simulink model "main_simulation"  (R2022b)
settings: Solver=VariableStepAuto  StartTime=0  StopTime=1372  FixedStep=0.1  MaxStep=0.1  RelTol=1e-3
values from neighbouring files (symbols this model uses):
  T = T(1:length(T)-100)    [data_loader.m]
libraries: spsVoltageMeasurementLib x2, spsControlledVoltageSourceLib x2, spsPMSynchronousMachineModel x1, simulink x1, autolibshared x1, slpidlib x1, spsStairGeneratorLib x1, spspowerguiLib x1
settings Model: Creator=Ahmad Hussain Safder  LastModifiedBy=safder.1
settings SolverCC: ZeroCrossAlgorithm=Adaptive
settings DataIOCC: SaveOutput=off  SaveTime=off  ReturnWorkspaceOutputs=off
settings DebuggingCC: IgnoredZcDiagnostic=none  UnconnectedInputMsg=warning  UnconnectedOutputMsg=warning  UnconnectedLineMsg=warning  ArithmeticOperatorsInVariantConditions=warning
settings ModelReferenceCC: EnableRefExpFcnMdlSchedulingChecks=on
settings SFSimCC: CustomCodeUndefinedFunction=UseInterfaceOnly

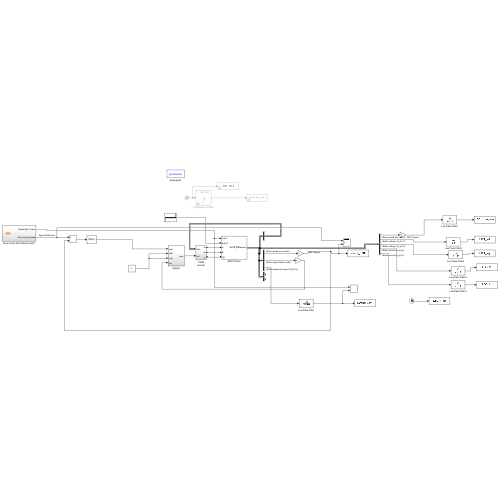
[thumbnail: Simulink's stored preview of the top-level diagram]
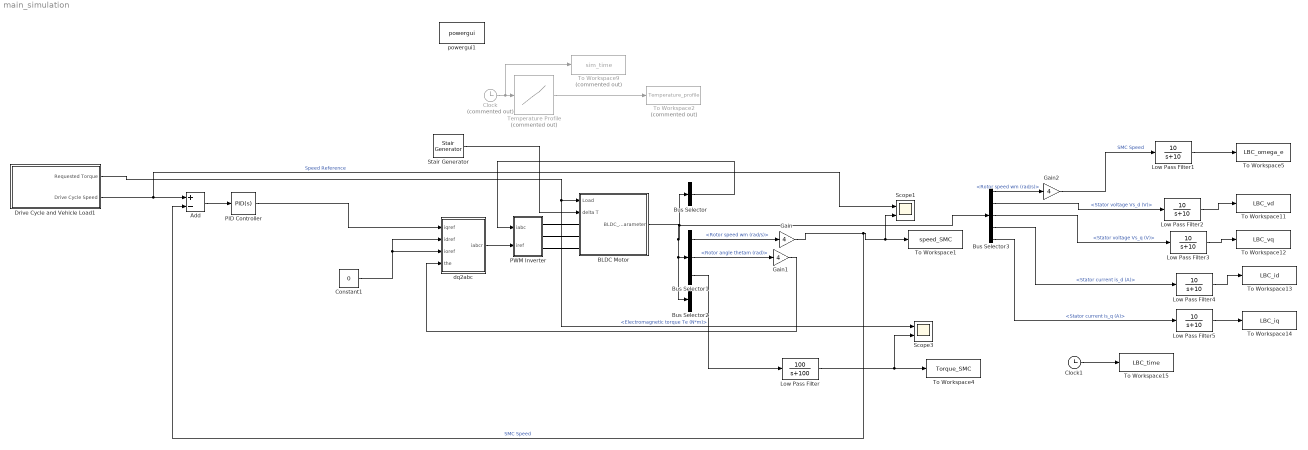
== system main_simulation ==
  Add : Sum  Inputs=+-
  BLDC Motor : Subsystem  mask{Rs=0.05, L=0.000795, Lq=0.0021, Ld=0.0016, Flux=0.192, p=4, J=0.011, Tf=0, F=0.001889, alpha_con=0.004, Tempi=25, Tempf=25}
      mask prompts: Rs "Phase Resistor (ohm)"; L "Armature Inductance (H)"; Lq "Lq (H)"; Ld "Ld (H)"; Flux "Flux Linkage"; p "Number of Poles"; J "Rotor Inertia (kgm^2)"; F "Viscous Coefficient (Nms)"; alpha_con "Temperature Coefficient (/C)"; Tempi "Initial Temperature (C)"; Tempf "Final Temperature (C)"
      mask Display: image('bldc-motor-controller-500x500.jpg');
  Bus Selector : BusSelector  OutputSignals=Stator current is_a (A),Stator current is_b (A),Stator current is_c (A)  OutputAsBus=on
  Bus Selector1 : BusSelector  OutputSignals=Rotor speed wm (rad/s),Rotor angle thetam (rad),Electromagnetic torque Te (N*m)
  Bus Selector2 : BusSelector  OutputSignals=Stator current is_d (A),Stator current is_q (A)
  Bus Selector3 : BusSelector  OutputSignals=Rotor speed wm (rad/s),Stator voltage Vs_d (V),Stator voltage Vs_q (V),Stator current is_d (A),Stator current is_q (A)
  Clock : Clock  Commented=on
  Clock1 : Clock
  Constant1 : Constant  Value=0
  Drive Cycle and Vehicle Load1 : Subsystem
  Gain : Gain  Gain=4  SaturateOnIntegerOverflow=on  OutDataTypeStr=Inherit: Same as input  ParamDataTypeStr=Inherit: Same as input
  Gain1 : Gain  Gain=4  SaturateOnIntegerOverflow=on  OutDataTypeStr=Inherit: Same as input  ParamDataTypeStr=Inherit: Same as input
  Gain2 : Gain  Gain=4  SaturateOnIntegerOverflow=on  OutDataTypeStr=Inherit: Same as input  ParamDataTypeStr=Inherit: Same as input
  Low Pass Filter : TransferFcn  Numerator=[100]  Denominator=[1 100]
  Low Pass Filter{1..5} (5 alike) : TransferFcn  Numerator=[10]  Denominator=[1 10]
  PID Controller : slpidlib/PID Controller  Controller=PID  Form=Parallel  TimeDomain=Continuous-time  UseExternalTs=off  SampleTime=-1  IntegratorMethod=Forward Euler  FilterMethod=Forward Euler  ControllerParametersSource=internal  P=40  I=3  UseKiTs=off  D=0  N=100  UseFilter=on  TunerSelectOption=Transfer Function Based (PID Tuner App)  InitialConditionSource=internal  InitialConditionForIntegrator=0  InitialConditionForFilter=0  DifferentiatorICPrevScaledInput=0  ExternalReset=none  TrackingMode=off  Kt=1  LimitOutput=off  SatLimitsSource=internal  UpperSaturationLimit=inf  LowerSaturationLimit=-inf  LinearizeAsGain=on  AntiWindupMode=none  Kb=1  LimitIntegrator=off  UpperIntegratorSaturationLimit=inf  LowerIntegratorSaturationLimit=-inf  POutMin=[]  POutMax=[]  IOutMin=[]  IOutMax=[]  DOutMin=[]  DOutMax=[]  NOutMin=[]  NOutMax=[]  SumOutMin=[]  SumOutMax=[]  SaturationOutMin=[]  SaturationOutMax=[]  PParamMin=[]  PParamMax=[]  IParamMin=[]  IParamMax=[]  DParamMin=[]  DParamMax=[]  NParamMin=[]  NParamMax=[]  KbParamMin=[]  KbParamMax=[]  KtParamMin=[]  KtParamMax=[]  KbOutMin=[]  KbOutMax=[]  KtOutMin=[]  KtOutMax=[]  IntegratorOutMin=[]  IntegratorOutMax=[]  FilterOutMin=[]  FilterOutMax=[]  SumI1OutMin=[]  SumI1OutMax=[]  SumI2OutMin=[]  SumI2OutMax=[]  SumI3OutMin=[]  SumI3OutMax=[]  SumI4OutMin=[]  SumI4OutMax=[]  SumDOutMin=[]  SumDOutMax=[]  DifferentiatorOutMin=[]  DifferentiatorOutMax=[]  FilterDiffOutCoefMin=[]  FilterDiffOutCoefMax=[]  ReciprocalOutMin=[]  ReciprocalOutMax=[]  SumDenOutMin=[]  SumDenOutMax=[]  SumNumOutMin=[]  SumNumOutMax=[]  DivideOutMin=[]  DivideOutMax=[]  UdiffTsProdOutMin=[]  UdiffTsProdOutMax=[]  NTsProdOutMin=[]  NTsProdOutMax=[]  UintegralTsProdOutMin=[]  UintegralTsProdOutMax=[]  UngainTsProdOutMin=[]  UngainTsProdOutMax=[]  ClampingZeroOutDataTypeStr=Inherit: Inherit via back propagation  ClampingZeroOutMin=[]  ClampingZeroOutMax=[]  FilterDenConstantOutDataTypeStr=Inherit: Inherit via back propagation  FilterDenConstantOutMin=[]  FilterDenConstantOutMax=[]  PCopyOutDataTypeStr=Inherit: Inherit via back propagation  PCopyOutMin=[]  PCopyOutMax=[]  NCopyOutDataTypeStr=Inherit: Inherit via back propagation  NCopyOutMin=[]  NCopyOutMax=[]  IntegratorContinuousStateAttributes=''  IntegratorStateMustResolveToSignalObject=off  IntegratorRTWStateStorageClass=Auto  FilterContinuousStateAttributes=''  FilterStateMustResolveToSignalObject=off  FilterRTWStateStorageClass=Auto  ParallelPVariant=InternalParameters  IdealPVariant=Disabled  IVariant=InternalParameters  DVariant=InternalParameters  IntegratorVariant=Continuous  SatVariant=Disabled  AWVariant=Passthrough  PCopyVariant=Disabled  TRVariant=Disabled  FdbkBlocksVariant=Forward  IdealPFdbkVariant=Disabled  SatFdbkVariant=Disabled  DerivativeFilterVariant=ContFilter  NVariant=InternalParameters  NCopyVariant=Disabled  FilterICVariant=InternalICsFilter  IntegratorICVariant=InternalICs  ExternalResetVariant=Disabled  TRSumVariant=Passthrough  SumFdbkVariant=Disabled  SumVariant=Sum_PID  TsampFilterVariant=InternalTs  TsampNgainVariant=Passthrough  TsampIntegralVariant=Passthrough  ExternalSaturationOutDataTypeStr=Inherit: Same as second input
  PWM Inverter : Subsystem
  Scope1 : Scope  NumInputPorts=2
  Scope3 : Scope  NumInputPorts=2
  Stair Generator : spsStairGeneratorLib/Stair Generator  t=[0 500 1000 ]  e=[0 25 50]  Ts=0
  Temperature Profile : Lookup_n-D  Commented=on  NumberOfTableDimensions=1  BreakpointsForDimension1=t  Table=T  InternalRulePriority=Speed  RndMeth=Simplest
  To Workspace1 : ToWorkspace  VariableName=speed_SMC  SampleTime=-1
      settings: Decimation=dec  Save2DSignal=2-D array (concatenate along first dimension)
  To Workspace11 : ToWorkspace  VariableName=LBC_vd  SampleTime=-1
      settings: Decimation=dec  Save2DSignal=2-D array (concatenate along first dimension)
  To Workspace12 : ToWorkspace  VariableName=LBC_vq  SampleTime=-1
      settings: Decimation=dec  Save2DSignal=2-D array (concatenate along first dimension)
  To Workspace13 : ToWorkspace  VariableName=LBC_id  SampleTime=-1
      settings: Decimation=dec  Save2DSignal=2-D array (concatenate along first dimension)
  To Workspace14 : ToWorkspace  VariableName=LBC_iq  SampleTime=-1
      settings: Decimation=dec  Save2DSignal=2-D array (concatenate along first dimension)
  To Workspace15 : ToWorkspace  VariableName=LBC_time  SampleTime=-1
      settings: Decimation=dec  Save2DSignal=2-D array (concatenate along first dimension)
  To Workspace2 : ToWorkspace  Commented=on  VariableName=Temperature_profile  SampleTime=-1
      settings: Decimation=dec  Save2DSignal=2-D array (concatenate along first dimension)
  To Workspace4 : ToWorkspace  VariableName=Torque_SMC  SampleTime=-1
      settings: Decimation=dec  Save2DSignal=2-D array (concatenate along first dimension)
  To Workspace5 : ToWorkspace  VariableName=LBC_omega_e  SampleTime=-1
      settings: Decimation=dec  Save2DSignal=2-D array (concatenate along first dimension)
  To Workspace9 : ToWorkspace  Commented=on  VariableName=sim_time  SampleTime=-1
      settings: Decimation=dec  Save2DSignal=2-D array (concatenate along first dimension)
  dq2abc : Subsystem
  powergui1 : spspowerguiLib/powergui  SimulationMode=Continuous  SampleTime=1e-5  frequency=60  Iterations=50  frequencyindice=0  Pbase=100e6  ErrMax=1e-4  UnitsV=kV  UnitsW=MW  buscounter=0  FunctionMessages=off  echomessages=off  EnableUseOfTLC=off  CurrentSourceSwitches=off  DisableSnubberDevices=off  DisableRonSwitches=off  DisableVfSwitches=off  DisplayEquations=off  AutomaticDiscreteSolvers=on  SolverType=Tustin/Backward Euler (TBE)  Interpol=off  ExternalGateDelay=off  methode=off  Ts=100  x0status=blocks  SPID=on  SwTol=0  HookPort=off  NonlinearTolerance=1e-4  nMaxIteration=100  ContinueOnMaxIteration=off  RestoreLinks=warning  ResistiveCurrentMeasurement=off  Frange=[0:2:500]  Ylog=off  Xlog=on  ShowGrid=off  save=off  variable=ZData  structure=0  ZoomFFT=on  StartTime=0.0  cycles=1  DisplayStyle=1  fundamental=60  FreqAxis=off  MaxFrequency=1000  frequencyindicesteady=1  RmsSteady=1  display=off
  wires:
  Bus Selector1/1 -> Gain/1  "<Rotor speed wm (rad/s)>"
  Bus Selector1/2 -> Gain1/1  "<Rotor angle thetam (rad)>"
  BLDC Motor/1(BLDC_Parameter) -> Bus Selector2/1, Bus Selector1/1, Bus Selector/1, Bus Selector3/1
  dq2abc/1(iabcr) -> PWM Inverter/2(iref)
  Gain1/1 -> dq2abc/4(the)
  Bus Selector/1 -> PWM Inverter/1(iabc)
  Gain/1 -> Add/2, Scope1/2, To Workspace1/1  "SMC Speed"
  Bus Selector1/3 -> Low Pass Filter/1  "<Electromagnetic torque Te (N*m)>"
  Low Pass Filter/1 -> Scope3/2, To Workspace4/1
  Clock/1 -> To Workspace9/1, Temperature Profile/1
  Temperature Profile/1 -> To Workspace2/1
  Stair Generator/1 -> BLDC Motor/2(delta T)
  Bus Selector3/1 -> Gain2/1  "<Rotor speed wm (rad/s)>"
  Clock1/1 -> To Workspace15/1
  Drive Cycle and Vehicle Load1/2(Drive Cycle Speed) -> Scope1/1, Add/1  "Speed Reference"
  Add/1 -> PID Controller/1
  Drive Cycle and Vehicle Load1/1(Requested Torque) -> Scope3/1, BLDC Motor/1(Load)
  PID Controller/1 -> dq2abc/1(iqref)
  Constant1/1 -> dq2abc/3(ioref), dq2abc/2(idref)
  Low Pass Filter1/1 -> To Workspace5/1
  Gain2/1 -> Low Pass Filter1/1  "SMC Speed"
  Low Pass Filter5/1 -> To Workspace14/1
  Low Pass Filter4/1 -> To Workspace13/1
  Low Pass Filter3/1 -> To Workspace12/1
  Low Pass Filter2/1 -> To Workspace11/1
  Bus Selector3/2 -> Low Pass Filter2/1  "<Stator voltage Vs_d (V)>"
  Bus Selector3/3 -> Low Pass Filter3/1  "<Stator voltage Vs_q (V)>"
  Bus Selector3/4 -> Low Pass Filter4/1  "<Stator current is_d (A)>"
  Bus Selector3/5 -> Low Pass Filter5/1  "<Stator current is_q (A)>"
  connections:
  BLDC Motor/LConn1 -- PWM Inverter/RConn1
  BLDC Motor/LConn2 -- PWM Inverter/RConn2
  PWM Inverter/RConn3 -- BLDC Motor/LConn3

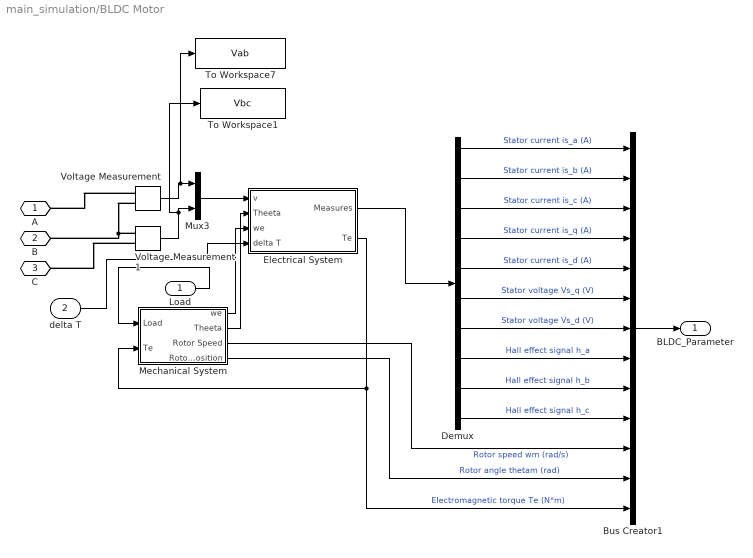
== system main_simulation/BLDC Motor ==
  Load : Inport
  delta T : Inport  Port=2
  Bus Creator1 : BusCreator  Inputs=13
  Demux : Demux  Outputs=[1,1,1,1,1,1,1,1,1,1]
  Electrical System : Subsystem
  Mechanical System : Subsystem
  Mux3 : Mux  Inputs=2
  To Workspace1 : ToWorkspace  VariableName=Vbc  SampleTime=-1
      settings: Decimation=dec  Save2DSignal=2-D array (concatenate along first dimension)
  To Workspace7 : ToWorkspace  VariableName=Vab  SampleTime=-1
      settings: Decimation=dec  Save2DSignal=2-D array (concatenate along first dimension)
  Voltage Measurement : spsVoltageMeasurementLib/Voltage Measurement  PhasorSimulation=off  OutputType=Complex  PSBequivalent=0
  Voltage Measurement1 : spsVoltageMeasurementLib/Voltage Measurement  PhasorSimulation=off  OutputType=Complex  PSBequivalent=0
  A : PMIOPort  Side=Left
  B : PMIOPort  Port=2  Side=Left
  C : PMIOPort  Port=3  Side=Left
  BLDC_Parameter : Outport  VectorParamsAs1DForOutWhenUnconnected=off
  wires:
  Voltage Measurement1/1 -> To Workspace1/1, Mux3/2
  Load/1 -> Mechanical System/1(Load)
  Mux3/1 -> Electrical System/1(v)
  Voltage Measurement/1 -> To Workspace7/1, Mux3/1
  Electrical System/2(Te) -> Bus Creator1/13, Mechanical System/2(Te)  "Electromagnetic torque Te (N*m)"
  Demux/9 -> Bus Creator1/9  "Hall effect signal h_b"
  Demux/6 -> Bus Creator1/6  "Stator voltage Vs_q (V)"
  Demux/10 -> Bus Creator1/10  "Hall effect signal h_c"
  Electrical System/1(Measures) -> Demux/1
  Demux/5 -> Bus Creator1/5  "Stator current is_d (A)"
  Demux/8 -> Bus Creator1/8  "Hall effect signal h_a"
  Demux/7 -> Bus Creator1/7  "Stator voltage Vs_d (V)"
  Bus Creator1/1 -> BLDC_Parameter/1
  Demux/1 -> Bus Creator1/1  "Stator current is_a (A)"
  Demux/2 -> Bus Creator1/2  "Stator current is_b (A)"
  Demux/3 -> Bus Creator1/3  "Stator current is_c (A)"
  Demux/4 -> Bus Creator1/4  "Stator current is_q (A)"
  Mechanical System/2(Theeta) -> Electrical System/2(Theeta)
  Mechanical System/3(Rotor Speed) -> Bus Creator1/11  "Rotor speed wm (rad/s)"
  Mechanical System/4(Rotor Position) -> Bus Creator1/12  "Rotor angle thetam (rad)"
  Mechanical System/1(we) -> Electrical System/3(we)
  delta T/1 -> Electrical System/4(delta T)
  connections:
  Voltage Measurement1/LConn1 -- Voltage Measurement/LConn2 -- B/RConn1
  Voltage Measurement/LConn1 -- A/RConn1
  Voltage Measurement1/LConn2 -- C/RConn1

== system main_simulation/Drive Cycle and Vehicle Load1 ==
  Drive Cycle Source : autolibshared/Drive Cycle Source  cycleVar=FTP72  fileVar=cycleFTP75.mat  tfinal="1372  seconds"  cycleRepeat=off  outAccPort=off  outGearPort=off  gearList=No gear data  t_wot1=5  xdot_woto=0  xdot_wot1=30  t_wot2=20  xdot_wot2=0  t_wotend=30  srcUnit=m/s  outUnit=m/s  srcAccUnit=m/s/s  outAccUnit=m/s^2  dt=0  aMode=1  faultOption=off  velBnd=2  velBndUnit=mph  inUnit=m/s  timeBnd=1  failOption=off  stopSim=off  maxFaultCnt=10  maxFaultTime=2  maxTotFaultTime=15  traceOption=off  dtTrace=1  traceWindow=10  lastDCname=FTP72  lastOutUnit=mph  lastDT=0  lastTB=1  lastSB=2  forceCalcBound=off
  Vehicle Loads : Subsystem
  Wheel Radius : Gain  Gain=(1/0.205)*(2)
  Wheel Radius1 : Gain  Gain=(0.205)*(1/10)
  Requested Torque : Outport
  Drive Cycle Speed : Outport  Port=2
  wires:
  Wheel Radius1/1 -> Requested Torque/1
  Wheel Radius/1 -> Drive Cycle Speed/1
  Vehicle Loads/1(F (N)) -> Wheel Radius1/1  "Vehicle_load (N)"
  Drive Cycle Source/1 -> Wheel Radius/1, Vehicle Loads/1(Vehicle Speed)

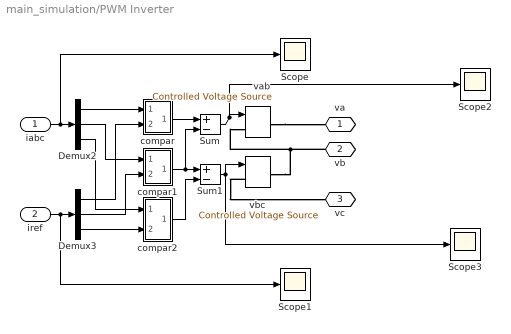
== system main_simulation/PWM Inverter ==
  iabc : Inport
  iref : Inport  Port=2
  Demux2 : Demux  Outputs=3
      settings: DisplayOption=none
  Demux3 : Demux  Outputs=3
      settings: DisplayOption=none
  Scope{,1..3} (4 alike) : Scope
  Sum : Sum  Inputs=+-  InputSameDT=on  SaturateOnIntegerOverflow=on  OutDataTypeStr=Inherit: Same as first input
  Sum1 : Sum  Inputs=+-  InputSameDT=on  SaturateOnIntegerOverflow=on  OutDataTypeStr=Inherit: Same as first input
  compar : Subsystem
  compar1 : Subsystem
  compar2 : Subsystem
  vab : spsControlledVoltageSourceLib/Controlled Voltage Source  Description=source block  Initialize=on  Source_Type=AC  Amplitude=0  Phase=0  Frequency=0  Measurements=None
      settings: AttributesFormatString=\n
  vbc : spsControlledVoltageSourceLib/Controlled Voltage Source  Description=source block  Initialize=on  Source_Type=AC  Amplitude=0  Phase=0  Frequency=0  Measurements=None
      settings: AttributesFormatString=\n
  va : PMIOPort  Side=Right
  vb : PMIOPort  Port=2  Side=Right
  vc : PMIOPort  Port=3  Side=Right
  wires:
  Demux3/3 -> compar2/2(icr)
  Demux3/2 -> compar1/2(ibr)
  Demux3/1 -> compar/2(iar)
  compar/1(va) -> Sum/1
  compar1/1(vb) -> Sum/2, Sum1/1
  compar2/1(vc) -> Sum1/2
  iabc/1 -> Scope/1, Demux2/1
  iref/1 -> Scope1/1, Demux3/1
  Sum/1 -> Scope2/1, vab/1
  Sum1/1 -> Scope3/1, vbc/1
  Demux2/2 -> compar1/1(ib)
  Demux2/1 -> compar/1(ia)
  Demux2/3 -> compar2/1(ic)
  connections:
  vab/RConn1 -- va/RConn1
  vb/RConn1 -- vab/LConn1 -- vbc/RConn1
  vbc/LConn1 -- vc/RConn1

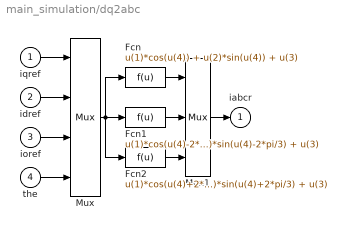
== system main_simulation/dq2abc ==
  iqref : Inport
  idref : Inport  Port=2
  ioref : Inport  Port=3
  the : Inport  Port=4
  Fcn : Fcn  Expr=u(1)*cos(u(4)) + u(2)*sin(u(4)) + u(3)
  Fcn1 : Fcn  Expr=u(1)*cos(u(4)-2*pi/3) + u(2)*sin(u(4)-2*pi/3) + u(3)
  Fcn2 : Fcn  Expr=u(1)*cos(u(4)+2*pi/3) + u(2)*sin(u(4)+2*pi/3) + u(3)
  Mux : Mux
  Mux1 : Mux  Inputs=3
  iabcr : Outport  InitialOutput=0  VectorParamsAs1DForOutWhenUnconnected=off
  wires:
  the/1 -> Mux/4
  ioref/1 -> Mux/3
  idref/1 -> Mux/2
  iqref/1 -> Mux/1
  Mux/1 -> Fcn1/1, Fcn2/1, Fcn/1
  Fcn1/1 -> Mux1/2
  Fcn/1 -> Mux1/1
  Fcn2/1 -> Mux1/3
  Mux1/1 -> iabcr/1

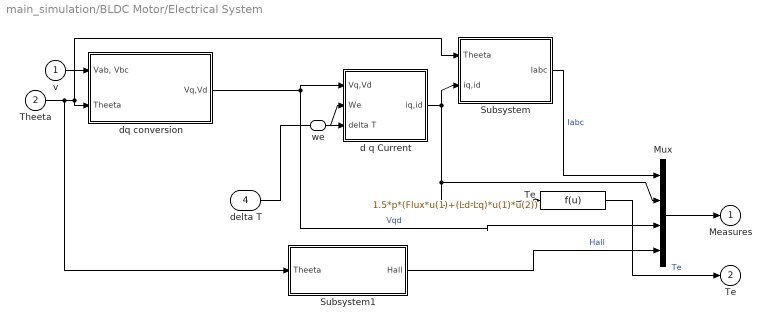
== system main_simulation/BLDC Motor/Electrical System ==
  v : Inport
  Theeta : Inport  Port=2
  we : Inport  Port=3
  delta T : Inport  Port=4
  Mux : Mux
  Subsystem : Subsystem
  Subsystem1 : Subsystem
  "Te " : Fcn  Expr=1.5*p*(Flux*u(1)+(Ld-Lq)*u(1)*u(2))
  d q Current : Subsystem
  dq conversion : Subsystem
  Measures : Outport  InitialOutput=0  VectorParamsAs1DForOutWhenUnconnected=off
  Te : Outport  Port=2  InitialOutput=0  VectorParamsAs1DForOutWhenUnconnected=off
  wires:
  Theeta/1 -> Subsystem1/1(Theeta), Subsystem/1(Theeta), dq conversion/2(Theeta)
  dq conversion/1(Vq,Vd) -> Mux/3, d q Current/1(Vq,Vd)  "Vqd"
  Mux/1 -> Measures/1
  Subsystem1/1(Hall) -> Mux/4  "Hall"
  "Te "/1 -> Te/1  "Te"
  d q Current/1(iq,id) -> Subsystem/2(iq,id), Mux/2, "Te "/1
  Subsystem/1(Iabc) -> Mux/1  "Iabc"
  v/1 -> dq conversion/1("Vab, Vbc")
  we/1 -> d q Current/2("We ")
  delta T/1 -> d q Current/3(delta T)

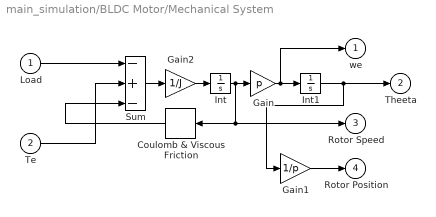
== system main_simulation/BLDC Motor/Mechanical System ==
  Load : Inport
  Te : Inport  Port=2
  Coulomb & Viscous Friction : simulink/Discontinuities/Coulomb & Viscous Friction  offset=Tf  gain=F
  Gain : Gain  Gain=p  SaturateOnIntegerOverflow=on  OutDataTypeStr=Inherit: Same as input  ParamDataTypeStr=Inherit: Same as input
  Gain1 : Gain  Gain=1/p
  Gain2 : Gain  Gain=1/J  SaturateOnIntegerOverflow=on  OutDataTypeStr=Inherit: Same as input  ParamDataTypeStr=Inherit: Same as input
  Int : Integrator
  Int1 : Integrator
  Sum : Sum  Inputs=-+-  InputSameDT=on  SaturateOnIntegerOverflow=on  OutDataTypeStr=Inherit: Same as first input
  we : Outport  InitialOutput=0  VectorParamsAs1DForOutWhenUnconnected=off
  Theeta : Outport  Port=2  InitialOutput=0  VectorParamsAs1DForOutWhenUnconnected=off
  Rotor Speed : Outport  Port=3  InitialOutput=0  VectorParamsAs1DForOutWhenUnconnected=off
  Rotor Position : Outport  Port=4  InitialOutput=0  VectorParamsAs1DForOutWhenUnconnected=off
  wires:
  Te/1 -> Sum/2
  Gain2/1 -> Int/1
  Load/1 -> Sum/1
  Coulomb & Viscous Friction/1 -> Sum/3
  Gain/1 -> we/1, Int1/1
  Sum/1 -> Gain2/1
  Int/1 -> Rotor Speed/1, Coulomb & Viscous Friction/1, Gain/1
  Int1/1 -> Gain1/1, Theeta/1
  Gain1/1 -> Rotor Position/1

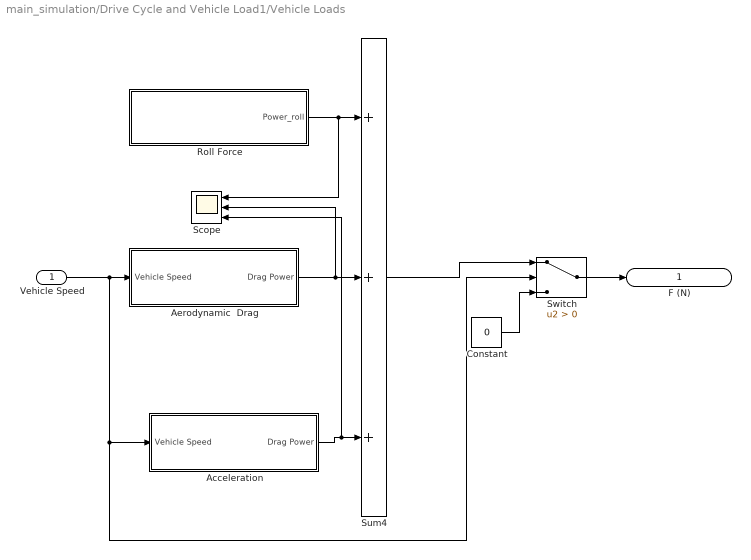
== system main_simulation/Drive Cycle and Vehicle Load1/Vehicle Loads ==
  Vehicle Speed : Inport
  "Acceleration " : Subsystem
  Aerodynamic  Drag : Subsystem
  Constant : Constant  Value=0
  Roll Force : Subsystem
  Scope : Scope  NumInputPorts=3
  Sum4 : Sum  Inputs=+++
  Switch : Switch  Criteria=u2 > Threshold  SaturateOnIntegerOverflow=off  InputSameDT=off
  F (N) : Outport  VectorParamsAs1DForOutWhenUnconnected=off
  wires:
  Aerodynamic  Drag/1(Drag Power) -> Scope/2, Sum4/2
  Roll Force/1(Power_roll) -> Scope/1, Sum4/1
  Vehicle Speed/1 -> Switch/2, "Acceleration "/1(Vehicle Speed), Aerodynamic  Drag/1(Vehicle Speed)
  "Acceleration "/1(Drag Power) -> Scope/3, Sum4/3
  Switch/1 -> F (N)/1
  Sum4/1 -> Switch/1
  Constant/1 -> Switch/3

== system main_simulation/PWM Inverter/compar ==
  ia : Inport
  iar : Inport  Port=2
  Relay1 : Relay  OnSwitchValue=0.05  OffSwitchValue=-0.05  OnOutputValue=300  OffOutputValue=-300
  Sum2 : Sum  Inputs=-+  InputSameDT=on  SaturateOnIntegerOverflow=on  OutDataTypeStr=Inherit: Same as first input
  Transfer Fcn : TransferFcn  Denominator=[5e-4 1]
  va : Outport  InitialOutput=0  VectorParamsAs1DForOutWhenUnconnected=off
  wires:
  iar/1 -> Sum2/2
  Sum2/1 -> Relay1/1
  Relay1/1 -> va/1
  ia/1 -> Transfer Fcn/1
  Transfer Fcn/1 -> Sum2/1

== system main_simulation/PWM Inverter/compar1 ==
  ib : Inport
  ibr : Inport  Port=2
  Relay1 : Relay  OnSwitchValue=0.05  OffSwitchValue=-0.05  OnOutputValue=300  OffOutputValue=-300
  Sum2 : Sum  Inputs=-+  InputSameDT=on  SaturateOnIntegerOverflow=on  OutDataTypeStr=Inherit: Same as first input
  Transfer Fcn : TransferFcn  Denominator=[5e-4 1]
  vb : Outport  InitialOutput=0  VectorParamsAs1DForOutWhenUnconnected=off
  wires:
  ibr/1 -> Sum2/2
  Sum2/1 -> Relay1/1
  Relay1/1 -> vb/1
  ib/1 -> Transfer Fcn/1
  Transfer Fcn/1 -> Sum2/1

== system main_simulation/PWM Inverter/compar2 ==
  ic : Inport
  icr : Inport  Port=2
  Relay1 : Relay  OnSwitchValue=0.05  OffSwitchValue=-0.05  OnOutputValue=300  OffOutputValue=-300
  Sum2 : Sum  Inputs=-+  InputSameDT=on  SaturateOnIntegerOverflow=on  OutDataTypeStr=Inherit: Same as first input
  Transfer Fcn : TransferFcn  Denominator=[5e-4 1]
  vc : Outport  InitialOutput=0  VectorParamsAs1DForOutWhenUnconnected=off
  wires:
  icr/1 -> Sum2/2
  Sum2/1 -> Relay1/1
  Relay1/1 -> vc/1
  ic/1 -> Transfer Fcn/1
  Transfer Fcn/1 -> Sum2/1

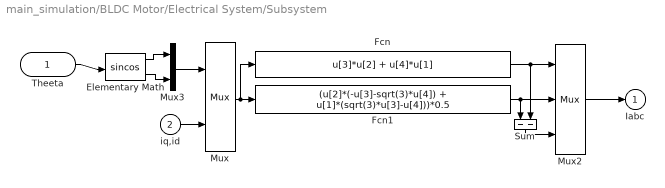
== system main_simulation/BLDC Motor/Electrical System/Subsystem ==
  Theeta : Inport
  iq,id : Inport  Port=2
  Elementary Math : Trigonometry  Operator=sincos
  Fcn : Fcn  Expr=u[3]*u[2] + u[4]*u[1]
  Fcn1 : Fcn  Expr=(u[2]*(-u[3]-sqrt(3)*u[4]) + u[1]*(sqrt(3)*u[3]-u[4]))*0.5
  Mux : Mux  Inputs=[2,2]
  Mux2 : Mux  Inputs=3
  Mux3 : Mux  Inputs=2
  Sum : Sum  Inputs=--  InputSameDT=on  SaturateOnIntegerOverflow=on  OutDataTypeStr=Inherit: Same as first input
  Iabc : Outport  InitialOutput=0  VectorParamsAs1DForOutWhenUnconnected=off
  wires:
  iq,id/1 -> Mux/2
  Theeta/1 -> Elementary Math/1
  Fcn/1 -> Sum/2, Mux2/1
  Mux/1 -> Fcn1/1, Fcn/1
  Sum/1 -> Mux2/3
  Mux2/1 -> Iabc/1
  Elementary Math/1 -> Mux3/1
  Elementary Math/2 -> Mux3/2
  Mux3/1 -> Mux/1
  Fcn1/1 -> Sum/1, Mux2/2

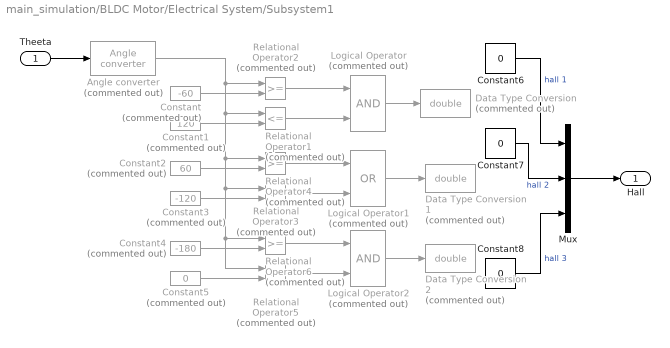
== system main_simulation/BLDC Motor/Electrical System/Subsystem1 ==
  Theeta : Inport
  Angle converter : spsPMSynchronousMachineModel/Continuous/Hall effect sensor/Angle converter  Commented=on  SystemSampleTime=-1  VariantActivationTime=update diagram  Latency=0  AutoFrameSizeCalculation=off
  Constant : Constant  Commented=on  Value=-60
  Constant1 : Constant  Commented=on  Value=120
  Constant2 : Constant  Commented=on  Value=60
  Constant3 : Constant  Commented=on  Value=-120
  Constant4 : Constant  Commented=on  Value=-180
  Constant5 : Constant  Commented=on  Value=0
  Constant6 : Constant  Value=0
  Constant7 : Constant  Value=0
  Constant8 : Constant  Value=0
  Data Type Conversion : DataTypeConversion  Commented=on  OutDataTypeStr=double
  Data Type Conversion1 : DataTypeConversion  Commented=on  OutDataTypeStr=double
  Data Type Conversion2 : DataTypeConversion  Commented=on  OutDataTypeStr=double
  Logical Operator : Logic  Commented=on  AllPortsSameDT=off  OutDataTypeStr=boolean
  Logical Operator1 : Logic  Commented=on  Operator=OR  AllPortsSameDT=off  OutDataTypeStr=boolean
  Logical Operator2 : Logic  Commented=on  AllPortsSameDT=off  OutDataTypeStr=boolean
  Mux : Mux  Inputs=3
  Relational Operator1 : RelationalOperator  Commented=on  Operator=<=
  Relational Operator2 : RelationalOperator  Commented=on
  Relational Operator3 : RelationalOperator  Commented=on  Operator=<=
  Relational Operator4 : RelationalOperator  Commented=on
  Relational Operator5 : RelationalOperator  Commented=on  Operator=<=
  Relational Operator6 : RelationalOperator  Commented=on
  Hall : Outport  VectorParamsAs1DForOutWhenUnconnected=off
  wires:
  Relational Operator6/1 -> Logical Operator2/1
  Constant1/1 -> Relational Operator1/2
  Logical Operator1/1 -> Data Type Conversion1/1
  Relational Operator4/1 -> Logical Operator1/1
  Constant4/1 -> Relational Operator6/2
  Angle converter/1 -> Relational Operator2/1, Relational Operator1/1, Relational Operator6/1, Relational Operator5/1, Relational Operator3/1, Relational Operator4/1
  Mux/1 -> Hall/1
  Relational Operator5/1 -> Logical Operator2/2
  Constant2/1 -> Relational Operator4/2
  Constant/1 -> Relational Operator2/2
  Constant5/1 -> Relational Operator5/2
  Theeta/1 -> Angle converter/1
  Relational Operator1/1 -> Logical Operator/2
  Logical Operator2/1 -> Data Type Conversion2/1
  Relational Operator2/1 -> Logical Operator/1
  Relational Operator3/1 -> Logical Operator1/2
  Logical Operator/1 -> Data Type Conversion/1
  Constant3/1 -> Relational Operator3/2
  Constant6/1 -> Mux/1  "hall 1"
  Constant7/1 -> Mux/2  "hall 2"
  Constant8/1 -> Mux/3  "hall 3"

== system main_simulation/BLDC Motor/Electrical System/d q Current ==
  Vq,Vd : Inport
  "We " : Inport  Port=2
  delta T : Inport  Port=3
  Demux : Demux  Outputs=2
  Mux : Mux  Inputs=2
  Subsystem : Subsystem
  Subsystem1 : Subsystem
  iq,id : Outport  InitialOutput=0  VectorParamsAs1DForOutWhenUnconnected=off
  wires:
  Mux/1 -> iq,id/1
  Demux/1 -> Subsystem/1(vq)
  "We "/1 -> Subsystem/2(we), Subsystem1/2(we)
  Demux/2 -> Subsystem1/3(vd)
  Vq,Vd/1 -> Demux/1
  Subsystem/1(iq) -> Subsystem1/1(iq), Mux/1
  Subsystem1/1(id) -> Subsystem/3(id), Mux/2
  delta T/1 -> Subsystem/4(delta T), Subsystem1/4(delta T)

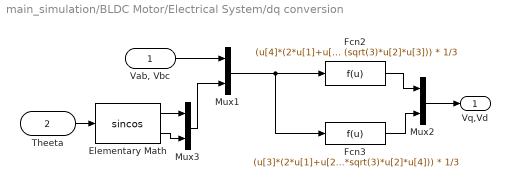
== system main_simulation/BLDC Motor/Electrical System/dq conversion ==
  "Vab, Vbc" : Inport
  Theeta : Inport  Port=2
  Elementary Math : Trigonometry  Operator=sincos
  Fcn2 : Fcn  Expr=(u[4]*(2*u[1]+u[2]) + (sqrt(3)*u[2]*u[3])) * 1/3
  Fcn3 : Fcn  Expr=(u[3]*(2*u[1]+u[2]) + (-1*sqrt(3)*u[2]*u[4])) * 1/3
  Mux1 : Mux  Inputs=[2 2]
  Mux2 : Mux  Inputs=2
  Mux3 : Mux  Inputs=2
  Vq,Vd : Outport  VectorParamsAs1DForOutWhenUnconnected=off
  wires:
  Mux1/1 -> Fcn3/1, Fcn2/1
  Elementary Math/2 -> Mux3/2
  Theeta/1 -> Elementary Math/1
  Mux3/1 -> Mux1/2
  Fcn3/1 -> Mux2/2
  Mux2/1 -> Vq,Vd/1
  "Vab, Vbc"/1 -> Mux1/1
  Fcn2/1 -> Mux2/1
  Elementary Math/1 -> Mux3/1

== system main_simulation/Drive Cycle and Vehicle Load1/Vehicle Loads/Acceleration  ==
  Vehicle Speed : Inport
  Constant1 : Constant  Value=350
  Gain : Gain  Gain=1/15
  Product : Product
  Drag Power : Outport  VectorParamsAs1DForOutWhenUnconnected=off
  wires:
  Vehicle Speed/1 -> Gain/1
  Constant1/1 -> Product/1
  Gain/1 -> Product/2
  Product/1 -> Drag Power/1

== system main_simulation/Drive Cycle and Vehicle Load1/Vehicle Loads/Aerodynamic  Drag ==
  Vehicle Speed : Inport
  Constant : Constant  Value=0.5
  Constant1 : Constant  Value=2.1
  Constant2 : Constant  Value=0.42
  Constant3 : Constant  Value=1.18
  Drag force =1/2*row_a*Cd*Af*v2 : Product  Inputs=5  RndMeth=Zero
  drag_v1 : Math  Operator=pow  SignedPower=on
  square : Constant  Value=2
  Drag Power : Outport  VectorParamsAs1DForOutWhenUnconnected=off
  wires:
  square/1 -> drag_v1/2
  Constant/1 -> Drag force =1/2*row_a*Cd*Af*v2/1
  drag_v1/1 -> Drag force =1/2*row_a*Cd*Af*v2/5
  Constant3/1 -> Drag force =1/2*row_a*Cd*Af*v2/4
  Constant2/1 -> Drag force =1/2*row_a*Cd*Af*v2/3
  Constant1/1 -> Drag force =1/2*row_a*Cd*Af*v2/2
  Drag force =1/2*row_a*Cd*Af*v2/1 -> Drag Power/1  "Drag_Force (N)"
  Vehicle Speed/1 -> drag_v1/1

== system main_simulation/Drive Cycle and Vehicle Load1/Vehicle Loads/Roll Force ==
  Constant : Constant  Value=0.013
  Constant1 : Constant  Value=350
  Constant2 : Constant  Value=9.8
  Roll_Force = Cr*M*g*cosd(road_grade) : Product  Inputs=3  RndMeth=Zero
  Power_roll : Outport  VectorParamsAs1DForOutWhenUnconnected=off
  wires:
  Roll_Force = Cr*M*g*cosd(road_grade)/1 -> Power_roll/1  "Roll_Force (N)"
  Constant/1 -> Roll_Force = Cr*M*g*cosd(road_grade)/1
  Constant1/1 -> Roll_Force = Cr*M*g*cosd(road_grade)/2
  Constant2/1 -> Roll_Force = Cr*M*g*cosd(road_grade)/3

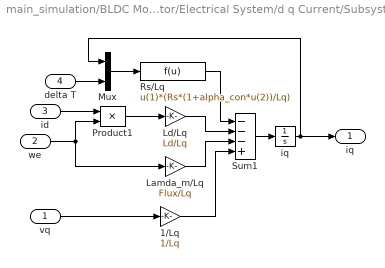
== system main_simulation/BLDC Motor/Electrical System/d q Current/Subsystem ==
  vq : Inport
  we : Inport  Port=2
  id : Inport  Port=3
  delta T : Inport  Port=4
  1/Lq : Gain  Gain=1/Lq  SaturateOnIntegerOverflow=on  OutDataTypeStr=Inherit: Same as input  ParamDataTypeStr=Inherit: Same as input
  Lamda_m/Lq : Gain  Gain=Flux/Lq  SaturateOnIntegerOverflow=on  OutDataTypeStr=Inherit: Same as input  ParamDataTypeStr=Inherit: Same as input
  Ld/Lq : Gain  Gain=Ld/Lq  SaturateOnIntegerOverflow=on  OutDataTypeStr=Inherit: Same as input  ParamDataTypeStr=Inherit: Same as input
  Mux : Mux  Inputs=2
  Product1 : Product  InputSameDT=on  SaturateOnIntegerOverflow=on  OutDataTypeStr=Inherit: Same as first input
  "Rs/Lq " : Fcn  Expr=u(1)*(Rs*(1+alpha_con*u(2))/Lq)
  Sum1 : Sum  Inputs=---+  InputSameDT=on  SaturateOnIntegerOverflow=on  OutDataTypeStr=Inherit: Same as first input
  "iq " : Integrator
  iq : Outport  InitialOutput=0  VectorParamsAs1DForOutWhenUnconnected=off
  wires:
  1/Lq/1 -> Sum1/4
  we/1 -> Product1/2, Lamda_m/Lq/1
  "iq "/1 -> Mux/1, iq/1
  Sum1/1 -> "iq "/1
  Product1/1 -> Ld/Lq/1
  id/1 -> Product1/1
  Lamda_m/Lq/1 -> Sum1/3
  Ld/Lq/1 -> Sum1/2
  vq/1 -> 1/Lq/1
  Mux/1 -> "Rs/Lq "/1
  delta T/1 -> Mux/2
  "Rs/Lq "/1 -> Sum1/1

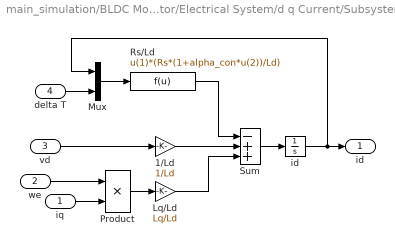
== system main_simulation/BLDC Motor/Electrical System/d q Current/Subsystem1 ==
  iq : Inport
  we : Inport  Port=2
  vd : Inport  Port=3
  delta T : Inport  Port=4
  1/Ld : Gain  Gain=1/Ld  SaturateOnIntegerOverflow=on  OutDataTypeStr=Inherit: Same as input  ParamDataTypeStr=Inherit: Same as input
  Lq/Ld : Gain  Gain=Lq/Ld  SaturateOnIntegerOverflow=on  OutDataTypeStr=Inherit: Same as input  ParamDataTypeStr=Inherit: Same as input
  Mux : Mux  Inputs=2
  Product : Product  InputSameDT=on  SaturateOnIntegerOverflow=on  OutDataTypeStr=Inherit: Same as first input
  "Rs/Ld " : Fcn  Expr=u(1)*(Rs*(1+alpha_con*u(2))/Ld)
  Sum : Sum  Inputs=-++  InputSameDT=on  SaturateOnIntegerOverflow=on  OutDataTypeStr=Inherit: Same as first input
  "id " : Integrator
  id : Outport  InitialOutput=0  VectorParamsAs1DForOutWhenUnconnected=off
  wires:
  Lq/Ld/1 -> Sum/3
  Sum/1 -> "id "/1
  vd/1 -> 1/Ld/1
  1/Ld/1 -> Sum/2
  Product/1 -> Lq/Ld/1
  iq/1 -> Product/2
  we/1 -> Product/1
  "id "/1 -> Mux/1, id/1
  delta T/1 -> Mux/2
  Mux/1 -> "Rs/Ld "/1
  "Rs/Ld "/1 -> Sum/1
